simulink model "all_in_one"  (R2021b)
settings: Solver=FixedStepAuto  StartTime=0.0  StopTime=StopTime  FixedStep=0.00005  RelTol=1e-3  EnableMultiTasking=on
PostLoadFcn:
  | st=1e6 ; dm=1e3 ; sf=0.5 ; df=0.3 ; dc=0.00001 ; dcr=0.001 ;
  | 
  | Kp=0.3 ; Ki=4.0 ; T=0.01 ;
  | 
  | [B,A]=butter(2,0.025) ; FF=tf(B,A,T) ;
undefined symbols (not defined in the file): AB, BC, CD, center, ee, EF, EG, front, gripper_base, gripper_finger_l, HF, kd_x, kd_y, kd_yaw, ki_x, ki_y, ki_yaw, kp_x, kp_y, kp_yaw, l1, l2, l3, link_dim, m1, m2, m3, m4, pin_r, rear, roll_x_offset, roll_y_offset, roll_z_offset, track_height, track_width, width_of_body, X, Y, Z
libraries: sm_lib x391, nesl_utility x30, slpidlib x3
(part 8 of 8)

== matlab function all_in_one/Manipulator control system/move comands ==
  data: p output; err_pose input; err_gripper input; cur_p input; grasp output; next_move output; cur_grasp input; cur_next_move input
function [p,grasp,next_move] = fcn(err_pose, err_gripper, cur_p, cur_grasp, cur_next_move)

body_error = 0.05; % Погрешность для перемещения робота
gripper_error = 0.01; % Погрешность позиционирования схвата
p = cur_p;
grasp = cur_grasp;
next_move = cur_next_move;

% Ожидаем прибытия в точку. Только по прибытию ( с указанной погрешностью)
% дается следующая точка и выполняются необходимые действия (команды для
% схвата)
if abs(err_pose(1)) <= body_error && abs(err_pose(2)) <= body_error && abs(err_pose(3)) <= body_error
    if (abs(err_gripper(1)) <= gripper_error && abs(err_gripper(2)) <= gripper_error && abs(err_gripper(3)) <= gripper_error)
        p = cur_p + 1;
        if cur_p == 1
        end
        if cur_p == 2
            grasp = 1;
            next_move = 1;
        end
        if cur_p == 4
            grasp = -1;
        end
    else
        p = cur_p;
    end
else
    p = cur_p;
end

== matlab function all_in_one/Move control/Law ==
  data: wxy input; vx input; u output; vy input
function u = fcn(wxy, vx, vy)
r = 0.09;
l = 0.38;
w = 0.215;
u = 1/r*[
    -l-w 1 -1; %FL
    l+w 1 1;   %FR
    w 1 -1;    %CR
    -w 1 1;    %CL
    l+w 1 -1;  %RR
    -l-w 1 1   %RL
    ]*[ wxy; vx; vy];

== matlab function all_in_one/Manipulator control system/Direct kinematics ==
  data: q1 input; p_act output; q2 input; q3 input; l1 input; l2 input; l3 input; ee input
function p_act = fcn(q1,q2,q3,l1,l2,l3,ee)
p_act = [
    -sin(q1)*((l3 + ee)*cos(q2+q3)+l2*cos(q2));
    cos(q1)*((l3 + ee)*cos(q2+q3)+l2*cos(q2));
    l1+(l3 + ee)*sin(q2+q3)+l2*sin(q2)];

== matlab function all_in_one/Manipulator control system/gravity compensation ==
  data: q_a input; tau output; l1 input; l2 input; l3 input; m1 input; m2 input; m3 input; ee input; m4 input
function tau = fcn(q_a,l1,l2,l3,m1,m2,m3,ee,m4)
q1 = [1 0 0]*q_a;
q2 = [0 1 0]*q_a;
q3 = [0 0 1]*q_a;

g=9.80665;%gravitation

N=[0;...
   0.5*g*l2*cos(q2)*(m2+m3+m4);
   0.5*g*(l3 + ee)*(m3+m4)*cos(q3)]; % gravity compensation

tau = N;

== matlab function all_in_one/robot/getYaw ==
  data: r output; p output; w input; y output; x input; y input; z input
function [r,p,y] = fcn(w,x,y,z)

rpy = quat2eul([w x y z]);
r = rpy(1);
p = rpy(2);
y = rpy(3);

== matlab function all_in_one/Manipulator control system/Impedance ==
  data: q_a input; tau_i output; dq_a input; p_d input; dp_d input; p_a input; l1 input; l2 input; l3 input; ee input
function tau_i = fcn(q_a, dq_a, p_d, dp_d, p_a, l1, l2, l3,ee)
q1 = [1 0 0]*q_a;
q2 = [0 1 0]*q_a;
q3 = [0 0 1]*q_a;
w1 = [1 0 0]*dq_a;
w2 = [0 1 0]*dq_a;
w3 = [0 0 1]*dq_a;



K=1500; D=1100; % control parameters

J=[-cos(q1)*(((l3 + ee) + ee)*cos(q2+q3)+l2*cos(q2)) sin(q1)*((l3 + ee)*sin(q2+q3)+l2*sin(q2)) (l3 + ee)*sin(q2+q3)*sin(q1);...
   -sin(q1)*((l3 + ee)*cos(q2+q3)+l2*cos(q2)) ((l3 + ee)*sin(q2+q3)+l2*sin(q2))*(2*sin(q1/2)^2-1) -(l3 + ee)*sin(q2+q3)*cos(q1);
   0 (l3 + ee)*cos(q2+q3)+l2*cos(q2) (l3 + ee)*cos(q2+q3)];% Jacobian

v=J*dq_a; % linear velicity of end-effector

F=K*(p_d-p_a)+D*(dp_d-v); % force
 tau_i=J.'*F; % impedance torque

== matlab function all_in_one/Move base targets ==
  data: n input; p output
function p = fcn(n)
if n == 0
    p = [0.95 0.8 0];
else
    p = [-0.95 -0.8 0];
end
